simulink model "unstable_system_attack"  (R2021a)
settings: Solver=VariableStepAuto  StartTime=0.0  StopTime=100  RelTol=1e-3
values from neighbouring files (symbols this model uses):
  sample_time = 1    [main1.m]    (also in main2.m)
libraries: commrandsrc3 x2, dspsrcs4 x1
settings Model: Creator=mehra  LastModifiedBy=mehra

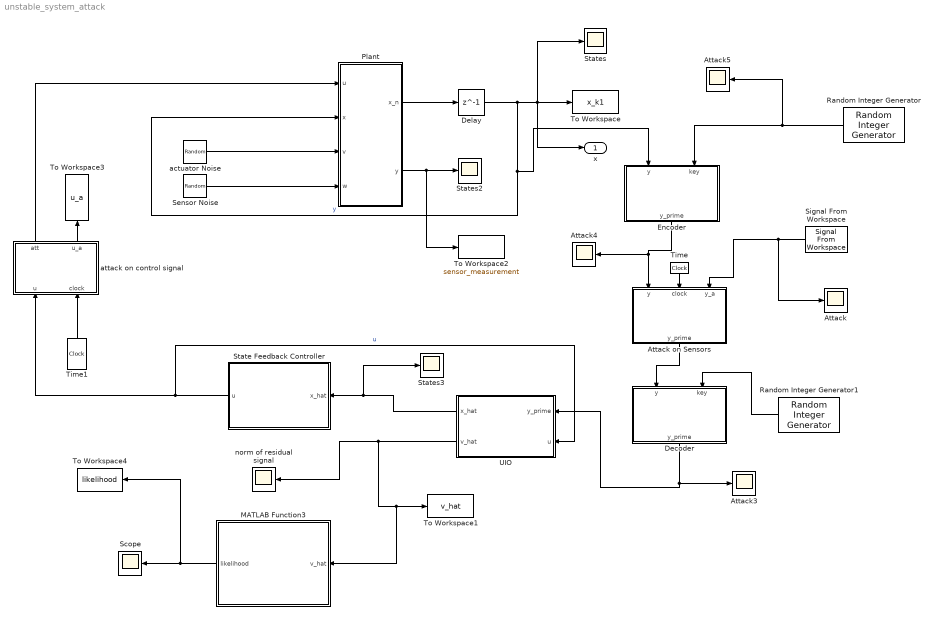
== system unstable_system_attack ==
  Attack{,3..5} (4 alike) : Scope
  Attack on Sensors : MATLAB Function  TreatAsAtomicUnit=on
  Decoder : MATLAB Function  TreatAsAtomicUnit=on
  Delay : Delay  DelayLength=1  InitialCondition=[0.1;0.1]  SampleTime=sample_time
  Encoder : MATLAB Function  TreatAsAtomicUnit=on
  MATLAB Function3 : MATLAB Function  TreatAsAtomicUnit=on
  Plant : MATLAB Function  TreatAsAtomicUnit=on
  Random Integer Generator : commrandsrc3/Random Integer Generator  SetSize=3  SeedSource=Parameter  Seed=20  SampleTime=sample_time  SamplesPerFrame=1  OutputDataType=double  SimulateUsing=Interpreted execution
  Random Integer Generator1 : commrandsrc3/Random Integer Generator  SetSize=3  SeedSource=Parameter  Seed=20  SampleTime=sample_time  SamplesPerFrame=1  OutputDataType=double  SimulateUsing=Interpreted execution
  Scope : Scope
  Sensor Noise : RandomNumber  Mean=[0 0]  Variance=[0.001 0.001]  Seed=[randi(100) randi(100)]  SampleTime=sample_time
  Signal From Workspace : dspsrcs4/Signal From Workspace  X=y_a  Ts=sample_time  nsamps=1  OutputAfterFinalValue=Cyclic repetition  ignoreOrWarnInputAndFrameLengths=off  OutputFrames=off
  State Feedback Controller : MATLAB Function  TreatAsAtomicUnit=on
  States : Scope
  States2 : Scope
  States3 : Scope
  Time : DigitalClock  SampleTime=sample_time
  Time1 : DigitalClock  SampleTime=sample_time
  To Workspace : ToWorkspace  VariableName=x_k1  SaveFormat=Timeseries  SampleTime=sample_time
  To Workspace1 : ToWorkspace  VariableName=v_hat  SaveFormat=Timeseries  SampleTime=sample_time
  To Workspace2 : ToWorkspace  VariableName=sensor_measurement  SaveFormat=Timeseries  SampleTime=sample_time
  To Workspace3 : ToWorkspace  VariableName=u_a  SaveFormat=Timeseries  SampleTime=sample_time
  To Workspace4 : ToWorkspace  VariableName=likelihood  SaveFormat=Timeseries  SampleTime=sample_time
  UIO : Subsystem
  actuator Noise : RandomNumber  Mean=[0 0]  Variance=[0.001 0.001]  Seed=[randi(100) randi(100)]  SampleTime=sample_time
  attack on control signal : MATLAB Function  TreatAsAtomicUnit=on
  norm of residual signal : Scope
  "x " : Outport  VectorParamsAs1DForOutWhenUnconnected=off
  wires:
  Plant/1(x_n) -> Delay/1
  Sensor Noise/1 -> Plant/4(w)
  Encoder/1(y_prime) -> Attack4/1, Attack on Sensors/1(y)
  Plant/2(y) -> To Workspace2/1, States2/1
  State Feedback Controller/1(u) -> attack on control signal/1(u), UIO/2(u)  "u"
  Decoder/1(y_prime) -> Attack3/1, UIO/1(y_prime)
  Delay/1 -> "x "/1, States/1, To Workspace/1, Plant/2(x), Encoder/1(y)  "y"
  Signal From Workspace/1 -> Attack on Sensors/3(y_a), Attack/1
  Attack on Sensors/1(y_prime) -> Decoder/1(y)
  actuator Noise/1 -> Plant/3(v)
  UIO/1(x_hat) -> States3/1, State Feedback Controller/1(x_hat)
  Time/1 -> Attack on Sensors/2(clock)
  attack on control signal/1(att) -> Plant/1(u)
  Time1/1 -> attack on control signal/2(clock)
  attack on control signal/2(u_a) -> To Workspace3/1
  UIO/2(v_hat) -> MATLAB Function3/1(v_hat), To Workspace1/1, norm of residual signal/1
  Random Integer Generator/1 -> Attack5/1, Encoder/2(key)
  Random Integer Generator1/1 -> Decoder/2(key)
  MATLAB Function3/1(likelihood) -> To Workspace4/1, Scope/1

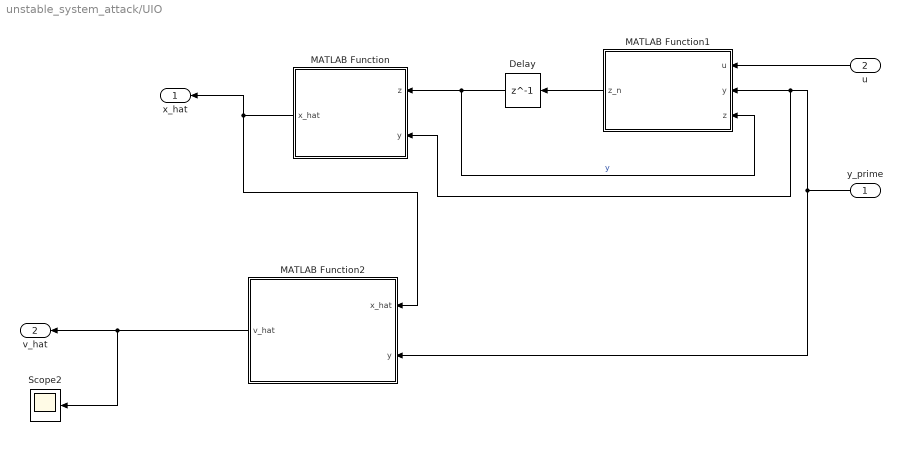
== system unstable_system_attack/UIO ==
  y_prime : Inport
  u : Inport  Port=2
  Delay : Delay  DelayLength=1  InitialCondition=zeros(2,1)  SampleTime=sample_time
  MATLAB Function : MATLAB Function  TreatAsAtomicUnit=on
  MATLAB Function1 : MATLAB Function  TreatAsAtomicUnit=on
  MATLAB Function2 : MATLAB Function  TreatAsAtomicUnit=on
  Scope2 : Scope
  x_hat : Outport  VectorParamsAs1DForOutWhenUnconnected=off
  v_hat : Outport  Port=2  VectorParamsAs1DForOutWhenUnconnected=off
  wires:
  MATLAB Function1/1(z_n) -> Delay/1
  u/1 -> MATLAB Function1/1(u)
  y_prime/1 -> MATLAB Function/2(y), MATLAB Function1/2(y), MATLAB Function2/2(y)
  Delay/1 -> MATLAB Function1/3(z), MATLAB Function/1(z)  "y"
  MATLAB Function/1(x_hat) -> x_hat/1, MATLAB Function2/1(x_hat)
  MATLAB Function2/1(v_hat) -> Scope2/1, v_hat/1

== matlab function unstable_system_attack/Plant ==
  data: x_n output; u input; y output; x input; v input; w input
function [x_n, y] = fcn(u, x, v, w)

%A=[1.0000    0.0001   -0.0010;0.5747    1.0000   -0.0003;0.0162    0.0000    1.0000];
%B = [0.1   -0.2; -0.0536    0.0332;0.1955   -0.5294];

A = [0.8 0; 
    0.5 1];
B = [1;
    0.5];
C = [2 0.5;
    0 1];
D = 0;

x_n = A*x + B*u + v;
y = C*x + D*u + w;

== matlab function unstable_system_attack/Attack on Sensors ==
  data: y input; y_prime output; clock input; y_a input
function y_prime = fcn(y, clock, y_a)
% this function should contain the attacker action on the sensor
% measurements
sigma1 = [2 -0.5;-0.5 1];
sigma2 = [1 -1;2 0];

% y_prime = y - y_a';
y_prime = y;
% 
end

== matlab function unstable_system_attack/State Feedback Controller ==
  data: x_hat input; u output
function u  = Controller(x_hat)
%two tanks model 



K = [0.1 -0.1];

u = K*x_hat;

== matlab function unstable_system_attack/MATLAB Function3 ==
  data: v_hat input; likelihood output
function likelihood = Anomaly_Detector(v_hat)

mu = -0.0011;
sigma = 0.0056;


likelihood = exp(-0.5*(v_hat(4:4)-mu')' * inv(sigma) * (v_hat(4:4)-mu'));

end

== matlab function unstable_system_attack/Encoder ==
  data: y input; y_prime output; key input
function y_prime = fcn(y,key)
% this function should contain the attacker action on the sensor
% measurements


% trans1 = [-0.547381274157748 0.836883349518582 ; 0.4 0.5];
% trans2 = [-0.547381274157748 0.836883349518582; 0.836883349518582 0.547381274157748];
% 
% trans1 = [-0.547381274157748 key;
%     -0.547381274157748 key];
% trans2 = [-0.547381274157748 0.836883349518582; 
%     0.836883349518582 0.547381274157748];
% 
% if key <= 1
%     y_prime = y'*trans1;
% else
%     y_prime = y'*trans2;
    
y_prime = y;
end

== matlab function unstable_system_attack/Decoder ==
  data: y input; y_prime output; key input
function y_prime = fcn(y,key)
% this function should contain the attacker action on the sensor
% measurements

% trans1 = [-0.547381274157748 0.836883349518582; 0.4 0.5];
% trans2 = [-0.547381274157748 0.836883349518582;0.836883349518582 0.547381274157748];

% trans1 = [-0.547381274157748 key;
%     -0.547381274157748 key];
% trans2 = [-0.547381274157748 0.836883349518582; 
%     0.836883349518582 0.547381274157748];
% 
% if key <= 1
%     y_prime = y*trans1';
% else
%     y_prime = y*trans2';
    
    y_prime = y;
end

== matlab function unstable_system_attack/UIO/MATLAB Function ==
  data: z input; x_hat output; y input
function x_hat = estimator(z,y)

M = [0.666666666666667,-0.666666666666667;
    0.666666666666667,-0.666666666666667];

x_hat = z + M*y;

== matlab function unstable_system_attack/UIO/MATLAB Function1 ==
  data: u input; z_n output; y input; z input
function z_n = UIO(u,y,z)

A = [0.8 0; 0.5 1];
B = [1;0.5];
C = [2 0.5;0 1];
D = 0;

M = [0.666666666666667,-0.666666666666667;
    0.666666666666667,-0.666666666666667];




L6 = [-0.0515    0.3474;
   -0.2058    1.3897];

z_n = (eye(2)-M*C)*(A*z + A*M*y+B*u) + L6*(y - C*z - C*M*y);

x_hat = z + M*y;

== matlab function unstable_system_attack/UIO/MATLAB Function2 ==
  data: x_hat input; v_hat output; y input
function v_hat = unknown_estimator(x_hat,y)

A = [0.8 0; 0.5 1];
B = [1;0.5];
C = [2 0.5;0 1];
% D = 0;

E = [1;1];
D = [zeros(2,2) eye(2,2)];
q = pinv(D)*y - pinv(D)*C*x_hat;
v_hat = q;

== matlab function unstable_system_attack/attack on control signal ==
  data: u input; att output; clock input; u_a output
function [att,u_a] = attack(u,clock)

att = u;
u_a = 1;
end
